simulink model "levitatore_sfun"  (R2017a)
settings: Solver=VariableStepAuto  StartTime=0.0  StopTime=50  RelTol=1e-3
values from neighbouring files (symbols this model uses):
  par = [m,km,R,L0,b,g]    [levitatoreMagnetico.m]    (also in temp1.mat = [0.2 19.62 50 0.5 0.1 9.81])
  ueq = 5    [levitatoreMagnetico.m]    (also in temp1.mat)
  xeq = [ueq/R*sqrt(km/m/g) 0 ueq/R]    [levitatoreMagnetico.m]    (also in temp1.mat = [0.316227766017 0 0.1])
libraries: cstblocks x1
settings Model: Creator=Enrico Donato  LastModifiedBy=Enrico Donato

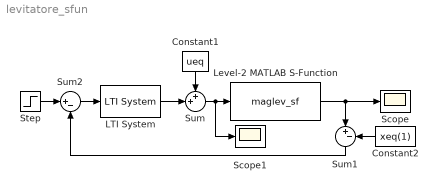
== system levitatore_sfun ==
  Constant1 : Constant  Value=ueq
  Constant2 : Constant  Value=xeq(1)
  LTI System : cstblocks/LTI System  sys=C1  IC=[]
  Level-2 MATLAB S-Function : M-S-Function  FunctionName=maglev_sf  Parameters=xeq,par
  Scope : Scope
  Scope1 : Scope
  Step : Step  Time=0  After=0.05  SampleTime=0
  Sum : Sum  Inputs=++|
  Sum1 : Sum  Inputs=|+-
  Sum2 : Sum  Inputs=|+-
  wires:
  Level-2 MATLAB S-Function/1 -> Sum1/1, Scope/1
  LTI System/1 -> Sum/2
  Sum/1 -> Scope1/1, Level-2 MATLAB S-Function/1
  Constant1/1 -> Sum/1
  Sum1/1 -> Sum2/2
  Sum2/1 -> LTI System/1
  Step/1 -> Sum2/1
  Constant2/1 -> Sum1/2
